simulink subsystem "fbw_transform_to_euler"  (R2020b)
settings: Solver=VariableStepAuto  StartTime=0.0  StopTime=10.0  RelTol=1e-3
libraries: simulink_extras x2
settings Model: Creator=Andreas  LastModifiedBy=Andreas

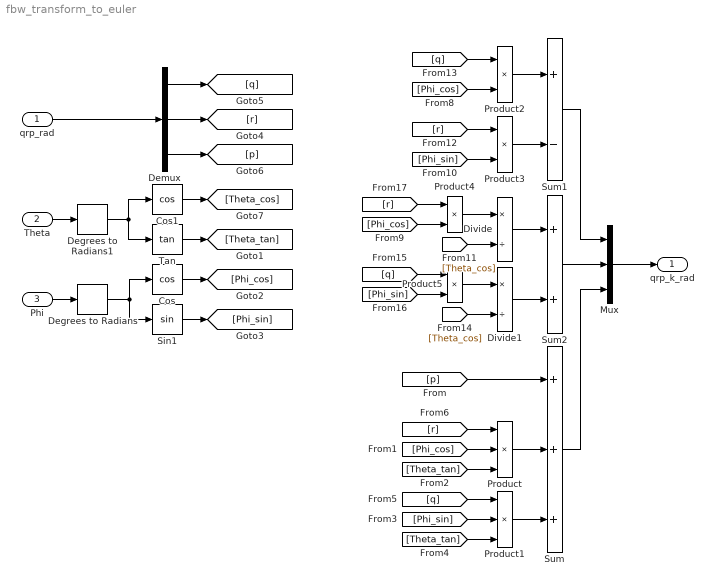
== system fbw_transform_to_euler ==
  qrp_rad : Inport
  Theta : Inport  Port=2
  Phi : Inport  Port=3
  Cos : Trigonometry  Operator=cos
  Cos1 : Trigonometry  Operator=cos
  Degrees to Radians : simulink_extras/Transformations/Degrees to Radians
  Degrees to Radians1 : simulink_extras/Transformations/Degrees to Radians
  Demux : Demux  Outputs=3
  Divide : Product  Inputs=*/
  Divide1 : Product  Inputs=*/
  Mux : Mux  Inputs=3
  Product : Product  Inputs=3
  Product1 : Product  Inputs=3
  Product{2..5} (4 alike) : Product
  Sin1 : Trigonometry
  Sum : Sum  Inputs=+++
  Sum1 : Sum  Inputs=+-
  Sum2 : Sum
  Tan : Trigonometry  Operator=tan
  qrp_k_rad : Outport
  wires:
  Theta/1 -> Degrees to Radians1/1
  Phi/1 -> Degrees to Radians/1
  Sum/1 -> Mux/3
  Tan/1 -> [Theta_tan]
  Demux/3 -> [p]
  Demux/1 -> [q]
  Sin1/1 -> [Phi_sin]
  Cos/1 -> [Phi_cos]
  [p] -> Sum/1
  Product/1 -> Sum/2
  Product1/1 -> Sum/3
  [Phi_cos] -> Product/2
  [Theta_tan] -> Product1/3
  [Phi_sin] -> Product1/2
  [Theta_tan] -> Product/3
  [r] -> Product/1
  [q] -> Product1/1
  [q] -> Product2/1
  Sum1/1 -> Mux/1
  Product3/1 -> Sum1/2
  Product2/1 -> Sum1/1
  [Phi_cos] -> Product2/2
  [Phi_sin] -> Product3/2
  [r] -> Product3/1
  [r] -> Product4/1
  Sum2/1 -> Mux/2
  Product4/1 -> Divide/1
  [Phi_cos] -> Product4/2
  [Theta_cos] -> Divide/2
  Divide/1 -> Sum2/1
  Product5/1 -> Divide1/1
  [q] -> Product5/1
  [Phi_sin] -> Product5/2
  [Theta_cos] -> Divide1/2
  Divide1/1 -> Sum2/2
  Cos1/1 -> [Theta_cos]
  Demux/2 -> [r]
  qrp_rad/1 -> Demux/1
  Mux/1 -> qrp_k_rad/1
  Degrees to Radians/1 -> Cos/1, Sin1/1
  Degrees to Radians1/1 -> Cos1/1, Tan/1
